simulink model "ECU_RCP"  (R2023b)
settings: Solver=FixedStepAuto  StartTime=0.0  StopTime=inf  FixedStep=TSample  RelTol=1e-3  EnableMultiTasking=on
values from neighbouring files (symbols this model uses):
  b_vkm = -10    [parameters.m]
  cM = 1/cn    (= 0.0328764778411)    [parameters.m]
  cphi = (phimax-phimin)/(phimaxV-phiminV)    (= 0.404635838948)    [parameters.m]
  iG = 18.125    [parameters.m]
  iG_car = [0.001 3.682 2.002 1.330 1.000 0.805]    [parameters.m]
  k1 = 0.5*c_W*A*p_L*1/(m_F+m_Zu)    (= 0.000412747747748)    [parameters.m]
  k2 = 0.0    (= 0)    [parameters.m]
  k3 = f_R*(m_F+m_Zu)*g*1/(m_F+m_Zu)    (= 0.0981)    [parameters.m]
  k4 = iD_car*eta/(r_stat*(m_F+m_Zu))    (= 0.00973685969564)    [parameters.m]
  k5 = 30*iD_car/(pi*r_dyn)    (= 108.639977642)    [parameters.m]
  m_vkm = -10/1000    (= -0.01)    [parameters.m]
  MFv = 0.4976    [parameters.m]
  p = [-5.1168e-6, 0.0518, 1.1411e+2]    [parameters.m]
  phi3_ref_idle = single(0.05)    [parameters.m]
  phimax = pi/2    (= 1.57079632679)    [parameters.m]
  phiminV = 0.5330    (= 0.533)    [parameters.m]
  RA = 2.579624359    [parameters.m]
  Ts_butter = 1/fs_butter    (= 0.01)    [parameters.m]
  UB = 15    [parameters.m]
  v_0 = 130/3.6    (= 36.1111111111)    [parameters.m]
undefined symbols (not defined in the file or in its folder): a_den_a_lim, a_den_stg, b_num_a_lim, b_num_stg, DiscIntNeverNeededParam, SampleTime, vel_profile
libraries: simulink x4, dspstat3 x1, slpidlib x1
settings Model: Creator=Sascha  LastModifiedBy=Sascha
settings SolverCC: PositivePriorityOrder=on  AutoInsertRateTranBlk=on
settings DataIOCC: ReturnWorkspaceOutputs=off
settings DebuggingCC: MergeDetectMultiDrivingBlocksExec=none
settings ModelReferenceCC: PropagateSignalLabelsOutOfModel=off
settings SFSimCC: SimCustomHeaderCode="#include \"profile_generator.h\""  SimUserIncludeDirs=..\Modules\
settings SFSimCC: SimUserSources=|
  | profile_generator.c
  | profile_generator_refac.c
settings RTWCC: RTWUseSimCustomCode=on  CustomHeaderCode="#include \"profile_generator.h\""  CustomInclude=..\Modules\  CodeExecutionProfiling=on  CodeProfilingSaveOptions=AllData
settings RTWCC: CustomSource=|
  | profile_generator.c
  | profile_generator_refac.c

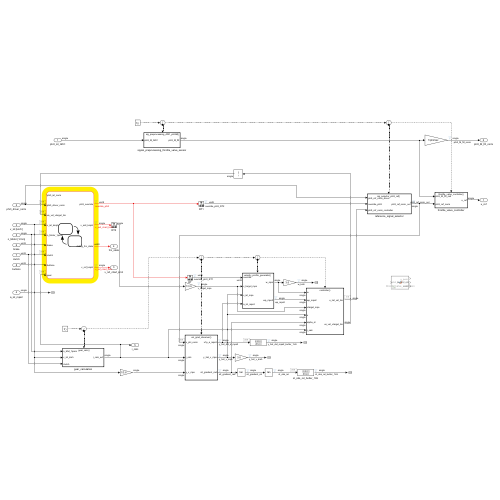
[thumbnail: Simulink's stored preview of the top-level diagram]
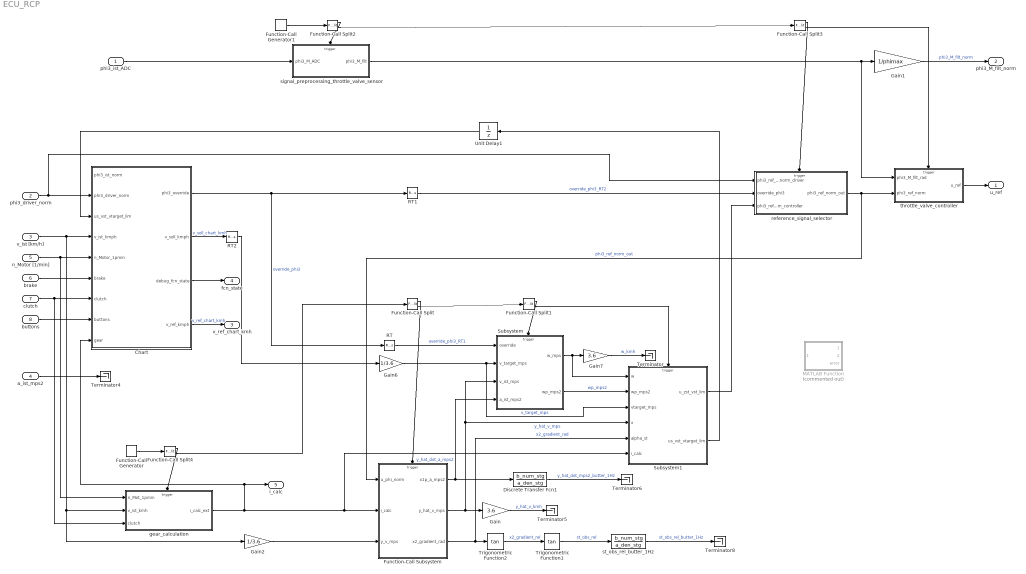
== system ECU_RCP ==
  phi3_ist_ADC : Inport  OutDataTypeStr=single
  phi3_driver_norm : Inport  Port=2  OutDataTypeStr=single
  v_ist [km/h] : Inport  Port=3  OutDataTypeStr=single
  a_ist_mps2 : Inport  Port=4  OutDataTypeStr=single
  n_Motor [1/min] : Inport  Port=5  OutDataTypeStr=single
  brake : Inport  Port=6  OutDataTypeStr=uint8
  clutch : Inport  Port=7  OutDataTypeStr=uint8
  buttons : Inport  Port=8  OutDataTypeStr=uint8
  Chart : Stateflow chart  TreatAsAtomicUnit=on
  Discrete Transfer Fcn1 : DiscreteTransferFcn  Numerator=b_num_stg  Denominator=a_den_stg  SampleTime=Ts_butter
  Function-Call Generator : simulink/Ports & Subsystems/Function-Call Generator  sample_time=0.005  numberOfIterations=1  DisallowWideOutput=off
  Function-Call Generator1 : simulink/Ports & Subsystems/Function-Call Generator  sample_time=0.001  numberOfIterations=1  DisallowWideOutput=off
  Function-Call Split{,1..4} (5 alike) : FunctionCallSplit  NumOutputPorts=2
  Function-Call Subsystem : Subsystem  TreatAsAtomicUnit=on
  Gain : Gain  Gain=3.6
  Gain1 : Gain  Gain=1/phimax
  Gain2 : Gain  Gain=1/3.6
  Gain6 : Gain  Gain=1/3.6
  Gain7 : Gain  Gain=3.6
  MATLAB Function : MATLAB Function  Commented=on  TreatAsAtomicUnit=on
  RT : RateTransition  OutPortSampleTime=0.005
  RT1 : RateTransition  OutPortSampleTime=0.001
  RT2 : RateTransition  OutPortSampleTime=0.005
  Subsystem : Subsystem  SystemSampleTime=0.01
  Subsystem1 : Subsystem
  Terminator{,4..6,8} (5 alike) : Terminator
  Trigonometric Function1 : Trigonometry  Operator=tan
  Trigonometric Function2 : Trigonometry  Operator=tan
  Unit Delay1 : UnitDelay  SampleTime=-1  HasFrameUpgradeWarning=on
  gear_calculation : Subsystem
  reference_signal_selector : Subsystem
  signal_preprocessing_throttle_valve_sensor : Subsystem
  st_obs_rel_butter_1Hz : DiscreteTransferFcn  Numerator=b_num_stg  Denominator=a_den_stg  SampleTime=Ts_butter
  throttle_valve_controller : Subsystem
  u_ref : Outport
  phi3_M_filt_norm : Outport  Port=2
  v_ref_chart_kmh : Outport  Port=3
  fcn_state : Outport  Port=4
  i_calc : Outport  Port=5
  wires:
  Chart/2(v_soll_kmph) -> RT2/1  "v_soll_chart_kmh"
  n_Motor [1/min]/1 -> gear_calculation/1(n_Mot_1pmin), Chart/5(n_Motor_1pmin)
  brake/1 -> Chart/6(brake)
  clutch/1 -> gear_calculation/3(clutch), Chart/7(clutch)
  phi3_driver_norm/1 -> reference_signal_selector/1(phi3_ref_norm_driver), Chart/2(phi3_driver_norm)
  Chart/1(phi3_override) -> RT/1, RT1/1  "override_phi3"
  buttons/1 -> Chart/8(buttons)
  Gain7/1 -> Terminator/1  "w_kmh"
  Gain2/1 -> Function-Call Subsystem/3(y_v_mps)
  Trigonometric Function1/1 -> st_obs_rel_butter_1Hz/1  "st_obs_rel"
  v_ist [km/h]/1 -> gear_calculation/2(v_ist_kmh), Gain2/1, Chart/4(v_ist_kmph)
  a_ist_mps2/1 -> Terminator4/1
  Gain1/1 -> phi3_M_filt_norm/1  "phi3_M_filt_norm"
  st_obs_rel_butter_1Hz/1 -> Terminator8/1  "st_obs_rel_butter_1Hz"
  Discrete Transfer Fcn1/1 -> Terminator6/1  "y_hat_dot_mps2_butter_1Hz"
  Chart/3(debug_fcn_state) -> fcn_state/1
  Subsystem/1(w_mps) -> Gain7/1, Subsystem1/1(w)
  RT/1 -> Subsystem/1(override)  "override_phi3_RT1"
  Function-Call Split/1 -> Function-Call Subsystem/Trigger
  Function-Call Subsystem/1(x1p_a_mps2) -> Subsystem/4(a_ist_mps2), Discrete Transfer Fcn1/1  "y_hat_dot_a_mps2"
  Function-Call Subsystem/2(y_hat_v_mps) -> Subsystem/3(v_ist_mps), Subsystem1/4(x), Gain/1  "y_hat_v_mps"
  Function-Call Subsystem/3(x2_gradient_rad) -> Subsystem1/5(alpha_st), Trigonometric Function2/1  "x2_gradient_rad"
  Gain/1 -> Terminator5/1  "y_hat_v_kmh"
  Trigonometric Function2/1 -> Trigonometric Function1/1  "x2_gradient_rel"
  Subsystem/2(wp_mps2) -> Subsystem1/2(wp_mps2)  "wp_mps2"
  Function-Call Split4/2 -> Function-Call Split/1
  Function-Call Split1/2 -> Subsystem1/Trigger
  Function-Call Split1/1 -> Subsystem/Trigger
  RT2/1 -> Gain6/1
  Function-Call Split/2 -> Function-Call Split1/1
  Gain6/1 -> Subsystem1/3(vtarget_mps), Subsystem/2(v_target_mps)  "v_target_mps"
  Subsystem1/2(us_vst_vtarget_lim) -> Unit Delay1/1
  Unit Delay1/1 -> Chart/3(us_vst_vtarget_lim)
  Chart/4(v_ref_kmph) -> v_ref_chart_kmh/1  "v_ref_chart_kmh"
  throttle_valve_controller/1(u_ref) -> u_ref/1
  signal_preprocessing_throttle_valve_sensor/1(phi3_M_filt) -> Gain1/1, throttle_valve_controller/1(phi3_M_filt_rad)
  phi3_ist_ADC/1 -> signal_preprocessing_throttle_valve_sensor/1(phi3_M_ADC)
  reference_signal_selector/1(phi3_ref_norm_out) -> throttle_valve_controller/2(phi3_ref_norm), Function-Call Subsystem/1(u_phi_norm)  "phi3_ref_norm_out"
  RT1/1 -> reference_signal_selector/2(override_phi3)  "override_phi3_RT2"
  Subsystem1/1(u_zst_vst_lim) -> reference_signal_selector/3(phi3_ref_norm_controller)
  Function-Call Generator1/1 -> Function-Call Split2/1
  Function-Call Split2/1 -> signal_preprocessing_throttle_valve_sensor/Trigger
  Function-Call Split3/1 -> reference_signal_selector/Trigger
  Function-Call Split2/2 -> Function-Call Split3/1
  Function-Call Split3/2 -> throttle_valve_controller/Trigger
  Function-Call Split4/1 -> gear_calculation/Trigger
  Function-Call Generator/1 -> Function-Call Split4/1
  gear_calculation/1(i_calc_ext) -> Chart/9(gear), i_calc/1, Subsystem1/6(i_calc), Function-Call Subsystem/2(i_calc)

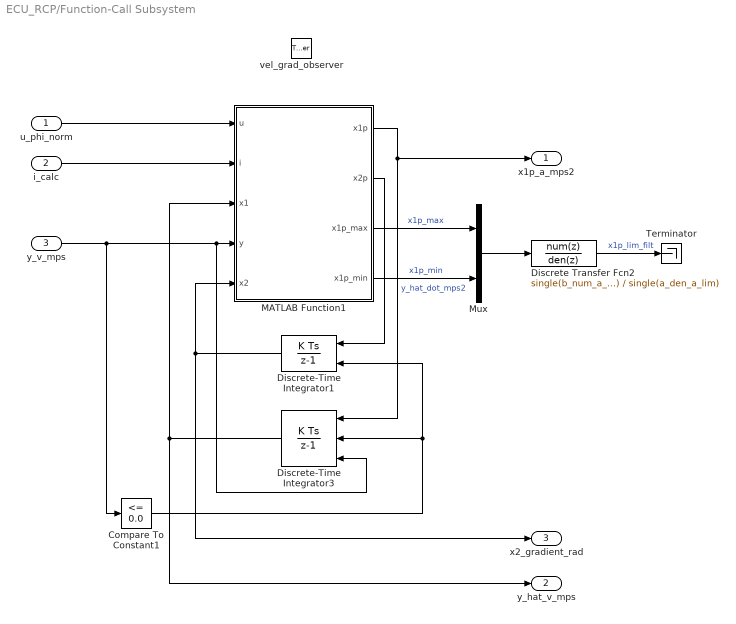
== system ECU_RCP/Function-Call Subsystem ==
  u_phi_norm : Inport  OutDataTypeStr=single
  i_calc : Inport  Port=2  OutDataTypeStr=single
  y_v_mps : Inport  Port=3  OutDataTypeStr=single
  vel_grad_observer : TriggerPort  TriggerType=function-call  VariantControl=(inherit)
  Compare To Constant1 : simulink/Logic and Bit Operations/Compare To Constant  relop=<=  const=0.0  OutDataTypeStr=boolean
  Discrete Transfer Fcn2 : DiscreteTransferFcn  Numerator=single(b_num_a_lim)  Denominator=single(a_den_a_lim)  InitialStates=single(0)
  Discrete-Time Integrator1 : DiscreteIntegrator  ExternalReset=sampled level  SampleTime=-1  LimitOutput=on  UpperSaturationLimit=0.4636  LowerSaturationLimit=-0.4636  ICPrevOutput=DiscIntNeverNeededParam  ICPrevScaledInput=DiscIntNeverNeededParam
  Discrete-Time Integrator3 : DiscreteIntegrator  ExternalReset=sampled level  InitialConditionSource=external  InitialCondition=v_0  SampleTime=-1  LimitOutput=on  UpperSaturationLimit=250/3.6  LowerSaturationLimit=0  ICPrevOutput=DiscIntNeverNeededParam  ICPrevScaledInput=DiscIntNeverNeededParam
  MATLAB Function1 : MATLAB Function  TreatAsAtomicUnit=on
  Mux : Mux  Inputs=2
  Terminator : Terminator
  x1p_a_mps2 : Outport  OutDataTypeStr=single
  y_hat_v_mps : Outport  Port=2  OutDataTypeStr=single
  x2_gradient_rad : Outport  Port=3  OutDataTypeStr=single
  wires:
  MATLAB Function1/2(x2p) -> Discrete-Time Integrator1/1
  u_phi_norm/1 -> MATLAB Function1/1(u)
  Discrete-Time Integrator1/1 -> x2_gradient_rad/1, MATLAB Function1/5(x2)
  y_v_mps/1 -> Compare To Constant1/1, Discrete-Time Integrator3/3, MATLAB Function1/4(y)
  MATLAB Function1/1(x1p) -> x1p_a_mps2/1, Discrete-Time Integrator3/1  "y_hat_dot_mps2"
  Discrete-Time Integrator3/1 -> y_hat_v_mps/1, MATLAB Function1/3(x1)
  i_calc/1 -> MATLAB Function1/2(i)
  Compare To Constant1/1 -> Discrete-Time Integrator1/2, Discrete-Time Integrator3/2
  MATLAB Function1/4(x1p_min) -> Mux/2  "x1p_min"
  MATLAB Function1/3(x1p_max) -> Mux/1  "x1p_max"
  Mux/1 -> Discrete Transfer Fcn2/1
  Discrete Transfer Fcn2/1 -> Terminator/1  "x1p_lim_filt"

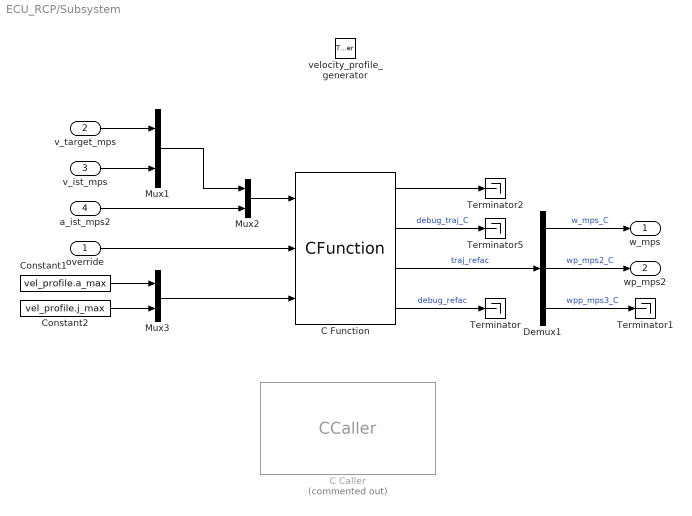
== system ECU_RCP/Subsystem ==
  override : Inport  OutDataTypeStr=uint8
  v_target_mps : Inport  Port=2
  v_ist_mps : Inport  Port=3
  a_ist_mps2 : Inport  Port=4
  velocity_profile_generator : TriggerPort  TriggerType=function-call  VariantControl=(inherit)
  C Caller : CCaller  Commented=on  FunctionName=profile_generator  PortSpecificationStruct="%)30     .    * <   8    (     @         %    \"     0    !     0         %  0 \"0    $    _    07)G3F%M90  4&]R=$YA;64 4V-O<&4     26YD97@     5'EP90      4VEZ90      27-';&]B86P   X    X    !@    @    $          4    (     0    8    !         !     &    =F5C7VEN   .    .     8    (    !          %    \"     $    &     0         0    !@   '9E8U]I;@  #@   #@    &    \"     0         !0    @    !   ...(+2085 chars)"  SampleTime=0.01
  C Function : CFunction  OutputCode=|  SampleTime=SampleTime  Ts=vel_profile.Ts  SampleTime=-1
      | params_t params;
      | params.t_s = Ts;
      | params.a_max = profile_params[0];
      | params.j_max = profile_params[1];
      | 
      | profile_generator(traj, debug, vec_in, override, &params);
      | 
      | profile_generator_refac(traj_refac, debug_refac, vec_in, override, &params);
  Constant1 : Constant  Value=vel_profile.a_max
  Constant2 : Constant  Value=vel_profile.j_max
  Demux1 : Demux  Outputs=3
  Mux1 : Mux  Inputs=2
  Mux2 : Mux  Inputs=2
  Mux3 : Mux  Inputs=2
  Terminator{,1..2,5} (4 alike) : Terminator
  w_mps : Outport
  wp_mps2 : Outport  Port=2
  wires:
  Mux1/1 -> Mux2/1
  v_ist_mps/1 -> Mux1/2
  v_target_mps/1 -> Mux1/1
  Mux2/1 -> C Function/1
  C Function/1 -> Terminator2/1
  Demux1/3 -> Terminator1/1  "wpp_mps3_C"
  Demux1/1 -> w_mps/1  "w_mps_C"
  Demux1/2 -> wp_mps2/1  "wp_mps2_C"
  override/1 -> C Function/2
  C Function/2 -> Terminator5/1  "debug_traj_C"
  Mux3/1 -> C Function/3
  Constant1/1 -> Mux3/1
  Constant2/1 -> Mux3/2
  a_ist_mps2/1 -> Mux2/2
  C Function/4 -> Terminator/1  "debug_refac"
  C Function/3 -> Demux1/1  "traj_refac"

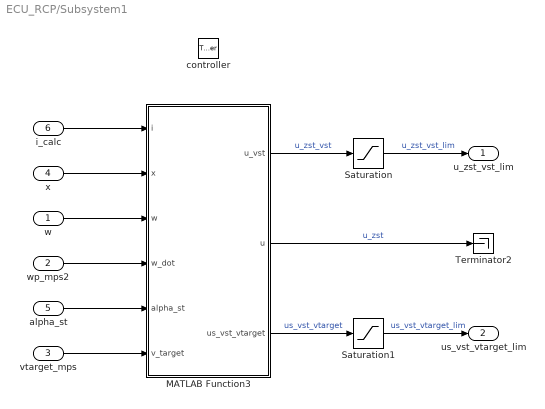
== system ECU_RCP/Subsystem1 ==
  w : Inport  OutDataTypeStr=single
  wp_mps2 : Inport  Port=2  OutDataTypeStr=single
  vtarget_mps : Inport  Port=3  OutDataTypeStr=single
  x : Inport  Port=4  OutDataTypeStr=single
  alpha_st : Inport  Port=5  OutDataTypeStr=single
  i_calc : Inport  Port=6  OutDataTypeStr=single
  controller : TriggerPort  TriggerType=function-call  VariantControl=(inherit)
  MATLAB Function3 : MATLAB Function  TreatAsAtomicUnit=on
  Saturation : Saturate  UpperLimit=1  LowerLimit=0
  Saturation1 : Saturate  UpperLimit=1  LowerLimit=0
  Terminator2 : Terminator
  u_zst_vst_lim : Outport  OutDataTypeStr=single
  us_vst_vtarget_lim : Outport  Port=2  OutDataTypeStr=single
  wires:
  wp_mps2/1 -> MATLAB Function3/4(w_dot)
  alpha_st/1 -> MATLAB Function3/5(alpha_st)
  i_calc/1 -> MATLAB Function3/1(i)
  MATLAB Function3/1(u_vst) -> Saturation/1  "u_zst_vst"
  Saturation/1 -> u_zst_vst_lim/1  "u_zst_vst_lim"
  MATLAB Function3/2(u) -> Terminator2/1  "u_zst"
  w/1 -> MATLAB Function3/3(w)
  x/1 -> MATLAB Function3/2(x)
  MATLAB Function3/3(us_vst_vtarget) -> Saturation1/1  "us_vst_vtarget"
  Saturation1/1 -> us_vst_vtarget_lim/1  "us_vst_vtarget_lim"
  vtarget_mps/1 -> MATLAB Function3/6(v_target)

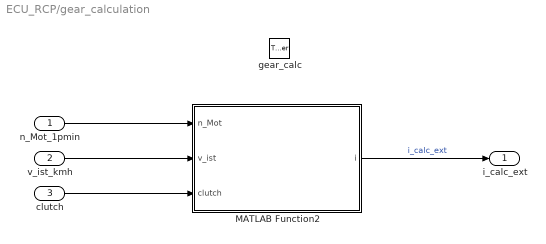
== system ECU_RCP/gear_calculation ==
  n_Mot_1pmin : Inport
  v_ist_kmh : Inport  Port=2
  clutch : Inport  Port=3
  gear_calc : TriggerPort  TriggerType=function-call  VariantControl=(inherit)
  MATLAB Function2 : MATLAB Function  TreatAsAtomicUnit=on
  i_calc_ext : Outport
  wires:
  MATLAB Function2/1(i) -> i_calc_ext/1  "i_calc_ext"
  clutch/1 -> MATLAB Function2/3(clutch)
  v_ist_kmh/1 -> MATLAB Function2/2(v_ist)
  n_Mot_1pmin/1 -> MATLAB Function2/1(n_Mot)

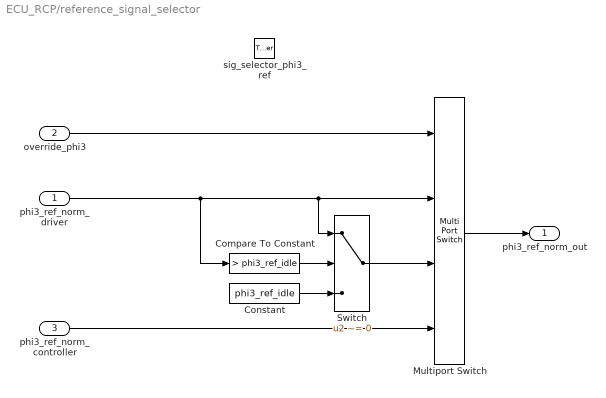
== system ECU_RCP/reference_signal_selector ==
  phi3_ref_norm_driver : Inport
  override_phi3 : Inport  Port=2
  phi3_ref_norm_controller : Inport  Port=3
  sig_selector_phi3_ref : TriggerPort  TriggerType=function-call  VariantControl=(inherit)
  Compare To Constant : simulink/Logic and Bit Operations/Compare To Constant  relop=>  const=phi3_ref_idle  OutDataTypeStr=boolean
  Constant : Constant  Value=phi3_ref_idle  OutDataTypeStr=single
  Multiport Switch : MultiPortSwitch  DataPortOrder=Zero-based contiguous  zeroidx=on  SaturateOnIntegerOverflow=off  InputSameDT=off
  Switch : Switch  Criteria=u2 ~= 0  SaturateOnIntegerOverflow=off  InputSameDT=off
  phi3_ref_norm_out : Outport
  wires:
  Multiport Switch/1 -> phi3_ref_norm_out/1
  phi3_ref_norm_controller/1 -> Multiport Switch/4
  override_phi3/1 -> Multiport Switch/1
  phi3_ref_norm_driver/1 -> Compare To Constant/1, Switch/1, Multiport Switch/2
  Compare To Constant/1 -> Switch/2
  Switch/1 -> Multiport Switch/3
  Constant/1 -> Switch/3

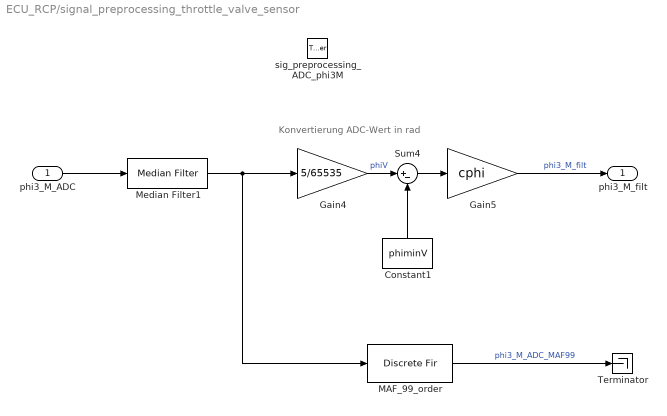
== system ECU_RCP/signal_preprocessing_throttle_valve_sensor ==
  note: Konvertierung ADC-Wert in rad
  phi3_M_ADC : Inport
  sig_preprocessing_ADC_phi3M : TriggerPort  TriggerType=function-call  VariantControl=(inherit)
  Constant1 : Constant  Value=phiminV  OutDataTypeStr=single
  Gain4 : Gain  Gain=5/65535
  Gain5 : Gain  Gain=cphi
  MAF_99_order : DiscreteFir  Coefficients=0.01*ones(1,100)
  Median Filter1 : dspstat3/Median Filter  WindowLength=5  SimulateUsing=Code generation
  Sum4 : Sum  Inputs=|+-
  Terminator : Terminator
  phi3_M_filt : Outport
  wires:
  Gain4/1 -> Sum4/1  "phiV"
  Median Filter1/1 -> MAF_99_order/1, Gain4/1
  Sum4/1 -> Gain5/1
  Gain5/1 -> phi3_M_filt/1  "phi3_M_filt"
  phi3_M_ADC/1 -> Median Filter1/1
  Constant1/1 -> Sum4/2
  MAF_99_order/1 -> Terminator/1  "phi3_M_ADC_MAF99"

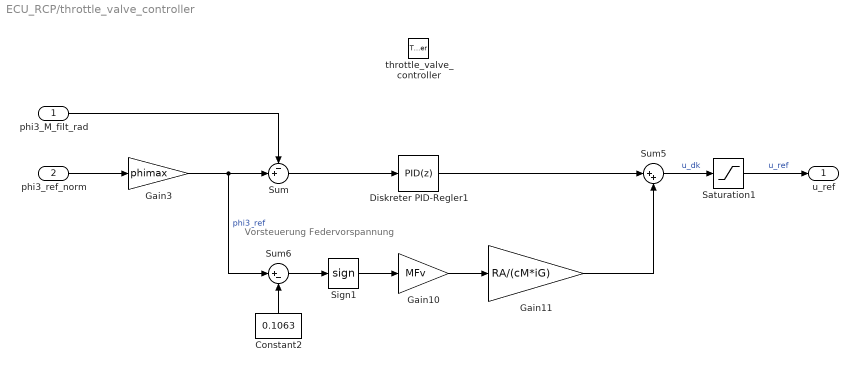
== system ECU_RCP/throttle_valve_controller ==
  note: Vorsteuerung Federvorspannung
  phi3_M_filt_rad : Inport
  phi3_ref_norm : Inport  Port=2
  throttle_valve_controller : TriggerPort  TriggerType=function-call  VariantControl=(inherit)
  Constant2 : Constant  Value=0.1063  OutDataTypeStr=single
  Diskreter PID-Regler1 : slpidlib/PID Controller  Controller=PID  Form=Ideal  TimeDomain=Discrete-time  UseExternalTs=off  SampleTime=-1  IntegratorMethod=Forward Euler  FilterMethod=Forward Euler  ControllerParametersSource=internal  P=29.8794278506843*1  I=0.464367214589814*2  UseKiTs=off  D=0.0103190181732761*2  N=2*358.825866890923  UseFilter=on  TunerSelectOption=Transfer Function Based (PID Tuner App)  InitialConditionSource=internal  InitialConditionForIntegrator=0  InitialConditionForFilter=0  DifferentiatorICPrevScaledInput=0  ExternalReset=none  TrackingMode=off  Kt=1  LimitOutput=on  SatLimitsSource=internal  UpperSaturationLimit=UB  LowerSaturationLimit=-UB  LinearizeAsGain=on  AntiWindupMode=clamping  Kb=1  LimitIntegrator=off  UpperIntegratorSaturationLimit=inf  LowerIntegratorSaturationLimit=-inf  POutMin=[]  POutMax=[]  IOutMin=[]  IOutMax=[]  DOutMin=[]  DOutMax=[]  NOutMin=[]  NOutMax=[]  SumOutMin=[]  SumOutMax=[]  SaturationOutMin=[]  SaturationOutMax=[]  PParamMin=[]  PParamMax=[]  IParamMin=[]  IParamMax=[]  DParamMin=[]  DParamMax=[]  NParamMin=[]  NParamMax=[]  KbParamMin=[]  KbParamMax=[]  KtParamMin=[]  KtParamMax=[]  KbOutMin=[]  KbOutMax=[]  KtOutMin=[]  KtOutMax=[]  IntegratorOutMin=[]  IntegratorOutMax=[]  FilterOutMin=[]  FilterOutMax=[]  SumI1OutMin=[]  SumI1OutMax=[]  SumI2OutMin=[]  SumI2OutMax=[]  SumI3OutMin=[]  SumI3OutMax=[]  SumI4OutMin=[]  SumI4OutMax=[]  SumDOutMin=[]  SumDOutMax=[]  DifferentiatorOutMin=[]  DifferentiatorOutMax=[]  FilterDiffOutCoefMin=[]  FilterDiffOutCoefMax=[]  ReciprocalOutMin=[]  ReciprocalOutMax=[]  SumDenOutMin=[]  SumDenOutMax=[]  SumNumOutMin=[]  SumNumOutMax=[]  DivideOutMin=[]  DivideOutMax=[]  UdiffTsProdOutMin=[]  UdiffTsProdOutMax=[]  NTsProdOutMin=[]  NTsProdOutMax=[]  UintegralTsProdOutMin=[]  UintegralTsProdOutMax=[]  UngainTsProdOutMin=[]  UngainTsProdOutMax=[]  ClampingZeroOutDataTypeStr=Inherit: Inherit via back propagation  ClampingZeroOutMin=[]  ClampingZeroOutMax=[]  FilterDenConstantOutDataTypeStr=Inherit: Inherit via back propagation  FilterDenConstantOutMin=[]  FilterDenConstantOutMax=[]  PCopyOutDataTypeStr=Inherit: Inherit via back propagation  PCopyOutMin=[]  PCopyOutMax=[]  NCopyOutDataTypeStr=Inherit: Inherit via back propagation  NCopyOutMin=[]  NCopyOutMax=[]  IntegratorContinuousStateAttributes=''  IntegratorStateMustResolveToSignalObject=off  IntegratorRTWStateStorageClass=Auto  FilterContinuousStateAttributes=''  FilterStateMustResolveToSignalObject=off  FilterRTWStateStorageClass=Auto  ParallelPVariant=Passthrough  IdealPVariant=InternalParameters  IVariant=InternalParameters  DVariant=InternalParameters  IntegratorVariant=Discrete  SatVariant=Enabled  AWVariant=DiscClampingIdeal  PCopyVariant=InternalParamsIdeal  TRVariant=Disabled  FdbkBlocksVariant=Forward  IdealPFdbkVariant=Disabled  SatFdbkVariant=Disabled  DerivativeFilterVariant=ForwardEulerFilter  NVariant=InternalParameters  NCopyVariant=Disabled  FilterICVariant=InternalICsFilter  IntegratorICVariant=InternalICs  ExternalResetVariant=Disabled  TRSumVariant=Passthrough  SumFdbkVariant=Disabled  SumVariant=Sum_PID  TsampFilterVariant=InternalTs  TsampNgainVariant=Passthrough  TsampIntegralVariant=Disabled_SignalSpec  ExternalSaturationOutDataTypeStr=Inherit: Same as second input
  Gain10 : Gain  Gain=MFv
  Gain11 : Gain  Gain=RA/(cM*iG)
  Gain3 : Gain  Gain=phimax
  Saturation1 : Saturate  UpperLimit=UB  LowerLimit=-UB
  Sign1 : Signum
  Sum : Sum  Inputs=-+|
  Sum5 : Sum  Inputs=|++
  Sum6 : Sum  Inputs=|+-
  u_ref : Outport
  wires:
  Sum/1 -> Diskreter PID-Regler1/1
  Sum6/1 -> Sign1/1
  Sum5/1 -> Saturation1/1  "u_dk"
  Diskreter PID-Regler1/1 -> Sum5/1
  Constant2/1 -> Sum6/2
  Gain3/1 -> Sum6/1, Sum/2  "phi3_ref"
  Gain11/1 -> Sum5/2
  Gain10/1 -> Gain11/1
  Sign1/1 -> Gain10/1
  phi3_ref_norm/1 -> Gain3/1
  Saturation1/1 -> u_ref/1  "u_ref"
  phi3_M_filt_rad/1 -> Sum/1

== matlab function ECU_RCP/Subsystem1/MATLAB Function3 ==
  data: k1 parameter; k2 parameter; k3 parameter; k4 parameter; k5 parameter; i input; p parameter; m_vkm parameter; b_vkm parameter; x input; iG_car parameter; w input; w_dot input; alpha_st input; u_vst output; u output; us_vst_vtarget output; v_target input
function [u_vst, u, us_vst_vtarget] = controller(k1, k2, k3, k4, k5, i, p, m_vkm, b_vkm, x, iG_car, w, w_dot, alpha_st, v_target)

if i ~= 0
    lam_des = -2;%-0.4;
    
    % xs = 130/3.6;
    xs = x;
    
    us = ((k1*xs^2+k2*xs+k3)*1/(k4*iG_car(i+1))-m_vkm*k5*iG_car(i+1)*xs-b_vkm)*1/(p(1)*k5^2*iG_car(i+1)^2*xs^2+p(2)*k5*iG_car(i+1)*xs+p(3));
    us_vst = ((k1*xs^2+k2*xs+k3+9.81*alpha_st)*1/(k4*iG_car(i+1))-m_vkm*k5*iG_car(i+1)*xs-b_vkm)*1/(p(1)*k5^2*iG_car(i+1)^2*xs^2+p(2)*k5*iG_car(i+1)*xs+p(3)); % Inkl. Vorsteuerung Steigung
    us_vst_vtarget = ((k1*v_target^2+k2*v_target+k3+9.81*alpha_st)*1/(k4*iG_car(i+1))-m_vkm*k5*iG_car(i+1)*v_target-b_vkm)*1/(p(1)*k5^2*iG_car(i+1)^2*v_target^2+p(2)*k5*iG_car(i+1)*v_target+p(3));
    
    a0 = -(-2*k1*xs-k2+2*k4*iG_car(i+1)^3*p(1)*k5^2*xs*us+k4*iG_car(i+1)^2*p(2)*k5*us+k4*iG_car(i+1)^2*m_vkm*k5);
    b = (k4*iG_car(i+1)^3*p(1)*k5^2*xs^2+k4*iG_car(i+1)^2*p(2)*k5*xs+k4*iG_car(i+1)*p(3));
    
    Dx = x - xs;
    Dw = w - xs;
    Dw_dot = w_dot;
    
    Du = ( Dw_dot - lam_des * Dw + (a0+lam_des) * Dx ) / b;
    
    u = Du + us;
    u_vst = Du + us_vst;
else
    u = single(0);
    u_vst = single(0);
    us_vst_vtarget = single(0);
end

== matlab function ECU_RCP/Function-Call Subsystem/MATLAB Function1 ==
  data: x1p output single; k1 parameter; k2 parameter; k3 parameter; k4 parameter; k5 parameter; u input single; i input; p parameter; m_vkm parameter; b_vkm parameter; x1 input single; iG_car parameter; y input single; x2p output single; x2 input single; x1p_max output single; x1p_min output single
function [x1p, x2p, x1p_max, x1p_min] = observer(k1, k2, k3, k4, k5, u, i, p, m_vkm, b_vkm, x1, iG_car, y, x2)

xs = x1; % Annahme nochmal hinterfagen!

if i ~= 0
    us = ((k1*xs^2+k2*xs+k3)*1/(k4*iG_car(i+1))-m_vkm*k5*iG_car(i+1)*xs-b_vkm)*1/(p(1)*k5^2*iG_car(i+1)^2*xs^2+p(2)*k5*iG_car(i+1)*xs+p(3));
    a0 = -(-2*k1*xs-k2+2*k4*iG_car(i+1)^3*p(1)*k5^2*xs*us+k4*iG_car(i+1)^2*p(2)*k5*us+k4*iG_car(i+1)^2*m_vkm*k5);
else
    a0 = -(-2*k1*xs-k2);
end

lam1d = -10;
lam2d = -10;

k1_obs = -lam1d-lam2d-a0;
k2_obs = -lam1d*lam2d/9.81;

y_hat = x1;

if i ~= 0
    x1p = -k1*x1^2-k2*x1-k3+k4*iG_car(i+1)*((p(1)*k5^2*iG_car(i+1)^2*x1^2+p(2)*k5*iG_car(i+1)*x1+p(3))*u+m_vkm*k5*iG_car(i+1)*x1+b_vkm) - 9.81*x2  + k1_obs*(y-y_hat);
    x1p_max = -k1*x1^2-k2*x1-k3+k4*iG_car(i+1)*((p(1)*k5^2*iG_car(i+1)^2*x1^2+p(2)*k5*iG_car(i+1)*x1+p(3))*1+m_vkm*k5*iG_car(i+1)*x1+b_vkm) - 9.81*x2  + k1_obs*(y-y_hat);
    x1p_min = -k1*x1^2-k2*x1-k3+k4*iG_car(i+1)*((p(1)*k5^2*iG_car(i+1)^2*x1^2+p(2)*k5*iG_car(i+1)*x1+p(3))*0+m_vkm*k5*iG_car(i+1)*x1+b_vkm) - 9.81*x2  + k1_obs*(y-y_hat);
else
    x1p = -k1*x1^2-k2*x1-k3 - 9.81*x2  + k1_obs*(y-y_hat);
    x1p_max = x1p;
    x1p_min = x1p;
end
x2p = k2_obs*(y-y_hat);

== stateflow chart ECU_RCP/Chart ==
  settings: updateMethod=DISCRETE  sampleTime=Ts_chart
  state Reset [commented out]
  state Drosselklappensteuerung [commented out]
    state manual_operation [commented out]
      en: phi3_override = 0;
      en: v_soll_kmph = v_ist_kmph;
      du: v_soll_kmph = v_ist_kmph;
      en: debug_fcn_state = 0;
    state velocity_control_override [commented out]
      state velocity_control [commented out]
        (history)
        state velocity_control_active [commented out]
          en: v_soll_kmph = v_ref_kmph;
          en: i1 = gear;
          du: i1 = gear;
          en: debug_fcn_state = 1;
        state rev_limiter_up [commented out]
          en: v_soll_kmph = v_lim_kmph;
          en: i2 = gear;
          du: i2 = gear;
          en: debug_fcn_state = 2;
          % [n_Motor_1pmin >= n_max_1pmin && i1 != 5]{v_lim_kmph = v_ist_kmph;}
        (default) -> Drosselklappensteuerung.velocity_control_override.velocity_control.velocity_control_active [commented out]
        Drosselklappensteuerung.velocity_control_override.velocity_control.velocity_control_active -> (junction 138) [commented out] : [i1!=0]
        (junction 138) -> Drosselklappensteuerung.velocity_control_override.velocity_control.rev_limiter_up [commented out] : [v_ref_kmph > v_lim_calc_kmph[i1-1] && i1 != 5]{v_lim_kmph = v_lim_calc_kmph[i1-1];}
        Drosselklappensteuerung.velocity_control_override.velocity_control.rev_limiter_up -> Drosselklappensteuerung.velocity_control_override.velocity_control.velocity_control_active [commented out] : [n_Motor_1pmin < n_max_1pmin && i1 < i2]
        (junction 136) -> Drosselklappensteuerung.velocity_control_override.velocity_control.velocity_control_active [commented out] : [v_ref_kmph < v_lim_calc_kmph[i2-1]]
        Drosselklappensteuerung.velocity_control_override.velocity_control.rev_limiter_up -> (junction 136) [commented out] : [i2!=0]
      state add1 [commented out]
      state driver_override [commented out]
        en: debug_fcn_state = 3;
      state clutch_pressed [commented out]
        en: phi3_override = 0;
        en: debug_fcn_state = 4;
      state add10 [commented out]
      state sub1 [commented out]
      state sub10 [commented out]
      state clutch_release [commented out]
      (default) -> Drosselklappensteuerung.velocity_control_override.velocity_control [commented out]
      Drosselklappensteuerung.velocity_control_override.velocity_control -> (junction 51) [commented out]
      (junction 54) -> Drosselklappensteuerung.velocity_control_override.velocity_control [commented out]
      Drosselklappensteuerung.velocity_control_override.velocity_control -> Drosselklappensteuerung.velocity_control_override.clutch_pressed [commented out] : [clutch == 1]{phi3_override = 0;}
      (junction 90) -> Drosselklappensteuerung.velocity_control_override.velocity_control [commented out] : [clutch == 0]{phi3_override = 1;}
      Drosselklappensteuerung.velocity_control_override.velocity_control -> Drosselklappensteuerung.velocity_control_override.driver_override [commented out] : [phi3_driver_norm >= 1.05*us_vst_vtarget_lim && phi3_driver_norm >= 0.02]{phi3_override = 0;}
      Drosselklappensteuerung.velocity_control_override.driver_override -> Drosselklappensteuerung.velocity_control_override.velocity_control [commented out] : [phi3_driver_norm <= 0.95*us_vst_vtarget_lim]{phi3_override = 1;}
      (junction 51) -> Drosselklappensteuerung.velocity_control_override.add1 [commented out] : [buttons == 1]
      Drosselklappensteuerung.velocity_control_override.add1 -> (junction 54) [commented out] : [buttons == 0]{v_ref_kmph = v_ref_kmph +1.0;}
      (junction 51) -> (junction 53) [commented out]
      (junction 55) -> (junction 54) [commented out]
      (junction 53) -> Drosselklappensteuerung.velocity_control_override.add10 [commented out] : [buttons == 2]
      Drosselklappensteuerung.velocity_control_override.add10 -> (junction 55) [commented out] : [buttons == 0]{v_ref_kmph = v_ref_kmph +10.0;}
      (junction 53) -> (junction 50) [commented out]
      (junction 56) -> (junction 55) [commented out]
      Drosselklappensteuerung.velocity_control_override.clutch_pressed -> Drosselklappensteuerung.velocity_control_override.clutch_release [commented out] : after(100,'msec')
      (junction 50) -> Drosselklappensteuerung.velocity_control_override.sub1 [commented out] : [buttons == 3]
      Drosselklappensteuerung.velocity_control_override.sub1 -> (junction 56) [commented out] : [buttons == 0]{v_ref_kmph = v_ref_kmph -1.0;}
      (junction 50) -> (junction 52) [commented out]
      (junction 57) -> (junction 56) [commented out]
      (junction 52) -> Drosselklappensteuerung.velocity_control_override.sub10 [commented out] : [buttons == 4]
      Drosselklappensteuerung.velocity_control_override.sub10 -> (junction 57) [commented out] : [buttons == 0]{v_ref_kmph = v_ref_kmph -10.0;}
      Drosselklappensteuerung.velocity_control_override.clutch_release -> (junction 90) [commented out]
    (default) -> Drosselklappensteuerung.manual_operation [commented out]
    Drosselklappensteuerung.manual_operation -> velocity_control_override [commented out] : [buttons>0 && buttons<5  && v_ist_kmph >= 20]{v_ref_kmph=v_ist_kmph; phi3_override = 1;}
    Drosselklappensteuerung.manual_operation -> velocity_control_override [commented out] : [buttons == 5 && v_ist_kmph >= 20]{v_ref_kmph=v_res_kmph; phi3_override = 1;}
    velocity_control_override -> Drosselklappensteuerung.manual_operation [commented out] : [buttons == 6 || brake == 1]{v_res_kmph = v_ref_kmph; phi3_override = 0;}
  state Reset1
  state Drosselklappensteuerung1
    state manual_operation
      en: phi3_override = 0;
      en: debug_fcn_state = 0;
    state engine_idle
    state velocity_control
      state velocity_control_active [parallel]
        settings: executionOrder=1
        state rev_limiter
          (history)
          state rev_limiter_passive
            en: v_soll_kmph = v_ref_kmph;
            du: v_soll_kmph = v_ref_kmph;
            en: debug_fcn_state = 1;
          state rev_limiter_up
            en: v_soll_kmph = state_machine_params.v_lim_calc_up_kmh[0][gear-1];
            en: i1 = gear;
            en: debug_fcn_state = 2;
          state rev_limiter_low
            en: v_soll_kmph = state_machine_params.v_lim_calc_low_kmh[0][gear-1];
            en: i1 = gear;
            en: debug_fcn_state = 2;
          (default) -> rev_limiter_passive
          rev_limiter_passive -> (junction 230) [order 1] : [gear != 0 && gear != 5]
          (junction 230) -> Drosselklappensteuerung1.velocity_control.velocity_control_active.rev_limiter.rev_limiter_up : [v_ref_kmph > state_machine_params.v_lim_calc_up_kmh[0][gear-1]]
          (junction 205) -> rev_limiter_passive : [v_ref_kmph < state_machine_params.v_lim_calc_up_kmh[0][gear-1]]
          Drosselklappensteuerung1.velocity_control.velocity_control_active.rev_limiter.rev_limiter_up -> (junction 205) [order 1] : [gear != 0]
          rev_limiter_passive -> (junction 326) [order 2] : [gear != 0]
          (junction 327) -> rev_limiter_passive : [v_ref_kmph > state_machine_params.v_lim_calc_low_kmh[0][gear-1]]
          Drosselklappensteuerung1.velocity_control.velocity_control_active.rev_limiter.rev_limiter_up -> Drosselklappensteuerung1.velocity_control.velocity_control_active.rev_limiter.rev_limiter_up [order 2] : [gear != i1]
          (junction 326) -> rev_limiter_low : [v_ref_kmph < state_machine_params.v_lim_calc_low_kmh[0][gear-1]]
          rev_limiter_low -> (junction 327) [order 1] : [gear != 0]
          rev_limiter_low -> rev_limiter_low [order 2] : [gear != i1]
        state driver_override
          en: debug_fcn_state = 3;
        state clutch_pressed
          en: phi3_override = 1;
          en: debug_fcn_state = 4;
        state clutch_release
        (default) -> rev_limiter
        rev_limiter -> Drosselklappensteuerung1.velocity_control.velocity_control_active.clutch_pressed [order 1] : [clutch == 1]{phi3_override = 1;}
        (junction 243) -> rev_limiter : [clutch == 0]{phi3_override = 2;}
        rev_limiter -> Drosselklappensteuerung1.velocity_control.velocity_control_active.driver_override [order 2] : [phi3_driver_norm >= 1.05*us_vst_vtarget_lim && phi3_driver_norm >= 0.02]{phi3_override = 0;}
        Drosselklappensteuerung1.velocity_control.velocity_control_active.driver_override -> rev_limiter : [phi3_driver_norm <= 0.95*us_vst_vtarget_lim]{phi3_override = 2;}
        Drosselklappensteuerung1.velocity_control.velocity_control_active.clutch_pressed -> Drosselklappensteuerung1.velocity_control.velocity_control_active.clutch_release : after(100,'msec')
        Drosselklappensteuerung1.velocity_control.velocity_control_active.clutch_release -> (junction 243)
      state button_analysis [parallel]
        settings: executionOrder=2
        state calc_v_ref
        state add1
        state add10
        state sub1
        state sub10
        (default) -> calc_v_ref
        calc_v_ref -> (junction 299)
        (junction 315) -> calc_v_ref
        (junction 299) -> Drosselklappensteuerung1.velocity_control.button_analysis.add1 [order 2] : [buttons == 1]
        Drosselklappensteuerung1.velocity_control.button_analysis.add1 -> (junction 280) : [buttons == 0]{v_ref_kmph = v_ref_kmph +1.0;}
        (junction 280) -> (junction 314)
        (junction 314) -> (junction 315) [order 1] : [v_ref_kmph > state_machine_params.v_ref_max]{v_ref_kmph = state_machine_params.v_ref_max;}
        (junction 299) -> (junction 287) [order 1]
        (junction 281) -> (junction 280)
        (junction 314) -> (junction 316) [order 2]
        (junction 317) -> (junction 315)
        (junction 287) -> Drosselklappensteuerung1.velocity_control.button_analysis.add10 [order 2] : [buttons == 2]
        Drosselklappensteuerung1.velocity_control.button_analysis.add10 -> (junction 281) : [buttons == 0]{v_ref_kmph = floor(v_ref_kmph/10.0)*10.0 + 10.0;}
        (junction 316) -> (junction 317) [order 1] : [v_ref_kmph < state_machine_params.v_ref_min]{v_ref_kmph = state_machine_params.v_ref_min;}
        (junction 287) -> (junction 282) [order 1]
        (junction 278) -> (junction 281)
        (junction 316) -> (junction 318) [order 2]
        (junction 320) -> (junction 317)
        (junction 282) -> Drosselklappensteuerung1.velocity_control.button_analysis.sub1 [order 2] : [buttons == 3]
        Drosselklappensteuerung1.velocity_control.button_analysis.sub1 -> (junction 278) : [buttons == 0]{v_ref_kmph = v_ref_kmph -1.0;}
        (junction 318) -> (junction 320)
        (junction 282) -> (junction 279) [order 1]
        (junction 296) -> (junction 278)
        (junction 279) -> Drosselklappensteuerung1.velocity_control.button_analysis.sub10 : [buttons == 4]
        Drosselklappensteuerung1.velocity_control.button_analysis.sub10 -> (junction 296) : [buttons == 0]{v_ref_kmph = ceil((v_ref_kmph)/10.0)*10.0 - 10.0;}
    (default) -> Drosselklappensteuerung1.manual_operation
    engine_idle -> Drosselklappensteuerung1.manual_operation : [clutch == 0 && gear != 0]{phi3_override = 0;}
    Drosselklappensteuerung1.manual_operation -> engine_idle [order 2] : [clutch == 1 || gear == 0]{phi3_override = 1;}
    Drosselklappensteuerung1.manual_operation -> (junction 334) [order 1] : [v_ist_kmph >= state_machine_params.v_ref_min && v_ist_kmph <= state_machine_params.v_ref_max && n_Motor_1pmin >= state_machine_params.n_Mot_min_1pmin]
    Drosselklappensteuerung1.velocity_control -> Drosselklappensteuerung1.manual_operation [order 1] : [buttons == 6 || brake == 1]{v_res_kmph = v_ref_kmph; phi3_override = 0;}
    Drosselklappensteuerung1.velocity_control -> Drosselklappensteuerung1.manual_operation [order 2] : [clutch == 0 && (gear == 0 || n_Motor_1pmin < (state_machine_params.n_Mot_min_1pmin - 200.0))]{v_res_kmph = v_ref_kmph; phi3_override = 0;}
    (junction 334) -> (junction 336) [order 2]
    (junction 334) -> Drosselklappensteuerung1.velocity_control [order 1] : [buttons>0 && buttons<5]{v_ref_kmph=v_ist_kmph; phi3_override = 2;}
    (junction 336) -> Drosselklappensteuerung1.velocity_control : [buttons == 5 && v_ref_kmph != 0.0]{v_ref_kmph=v_res_kmph; phi3_override = 2;}
  (default) -> Reset [commented out]
  (default) -> Reset1
  Reset -> Drosselklappensteuerung [commented out]
  Reset1 -> Drosselklappensteuerung1
  data: phi3_ist_norm input single; phi3_driver_norm input single; us_vst_vtarget_lim input single; v_ist_kmph input single; n_Motor_1pmin input single; brake input uint8; clutch input uint8; buttons input uint8; gear input single; phi3_override output uint8; v_soll_kmph output single; i1 local single; v_lim_kmph local single; v_res_kmph local single; debug_fcn_state output uint8; v_ref_kmph output single; state_machine_params parameter

== matlab function ECU_RCP/MATLAB Function ==
  data: u_pwm output; phi3_M_ADC_MAF99 input single; param_out output single; error output boolean; valve_calib parameter
function [u_pwm, param_out, error]  = throttle_valve_calibration(phi3_M_ADC_MAF99, valve_calib)
    persistent t
    if isempty(t)
        t = single(0.0);
    end

    param_out = single([0.0 0.0 0.0]);
    error = boolean(false);

    if t == 0.1
        if phi3_M_ADC_MAF99 >= valve_calib.phi_nop(1) && phi3_M_ADC_MAF99 <= valve_calib.phi_nop(3)
            param_out(2) = phi3_M_ADC_MAF99;
        else
            param_out(2) = valve_calib.phi_nop(2);
            error = boolean(true);
        end
    elseif t < 0.3
        if phi3_M_ADC_MAF99 >= valve_calib.phi_min(1) && phi3_M_ADC_MAF99 <= valve_calib.phi_min(3)
            param_out(1) = phi3_M_ADC_MAF99;
        else
            param_out(1) = valve_calib.phi_min(2);
            error = boolean(true);
        end
    elseif t < 0.5
        if phi3_M_ADC_MAF99 >= valve_calib.phi_max(1) && phi3_M_ADC_MAF99 <= valve_calib.phi_max(3)
            param_out(2) = phi3_M_ADC_MAF99;
        else
            param_out(2) = valve_calib.phi_max(2);
            error = boolean(true);
        end
    else
    end

end

== matlab function ECU_RCP/gear_calculation/MATLAB Function2 ==
  data: n_Mot input single; i output single; v_ist input single; clutch input; gear_calc_params parameter
function i = gear_calculation(n_Mot, v_ist, clutch, gear_calc_params)
    n_Getriebe_in_1pmin = n_Mot;
    n_Getriebe_out_1pmin = v_ist/(gear_calc_params.r_dyn*0.001*60*2*pi)*gear_calc_params.i_diff;
     
    if n_Getriebe_in_1pmin > 0 && n_Getriebe_out_1pmin > 0 && clutch == 0
        i_calc = n_Getriebe_in_1pmin/n_Getriebe_out_1pmin;
        
        if i_calc <= gear_calc_params.iG_car_up(5) && i_calc >= gear_calc_params.iG_car_low(5)
            i = single(5);
        elseif i_calc <= gear_calc_params.iG_car_up(4) && i_calc >= gear_calc_params.iG_car_low(4)
            i = single(4);
        elseif i_calc <= gear_calc_params.iG_car_up(3) && i_calc >= gear_calc_params.iG_car_low(3)
            i = single(3);
        elseif i_calc <= gear_calc_params.iG_car_up(2) && i_calc >= gear_calc_params.iG_car_low(2)
            i = single(2);
        elseif i_calc <= gear_calc_params.iG_car_up(1) && i_calc >= gear_calc_params.iG_car_low(1)
            i = single(1);
        else
            i = single(0);
        end
    
    else
        i = single(0);
    end
